simulink model "blance_robot"  (R2024a)
settings: Solver=ode15s  StartTime=0.0  StopTime=15  FixedStep=0.0025  RelTol=1e-3
values from neighbouring files (symbols this model uses):
  K_cons = [-4.92635870386 -6.18040077772 -1.81074270733 -1.19207999822 -32.1009473092 -3.5760389828 4.18688097447 0.16514939939 0.944125254207 0.571537384386 -4.92635870394 -6.18040077751 ... (240 elements, 40x6)]    [K_cons.mat]    (also in k_calc.m = zeros(40,6))
  X = [x1, x2, x1sq, x2sq, x1x2]    [k_calc.m]
undefined symbols (not defined in the file or in its folder): Y, Z
libraries: sm_lib x148, nesl_utility x26, slpidlib x3
(part 1 of 4)
settings Model: Creator=zhuho  LastModifiedBy=zhuho

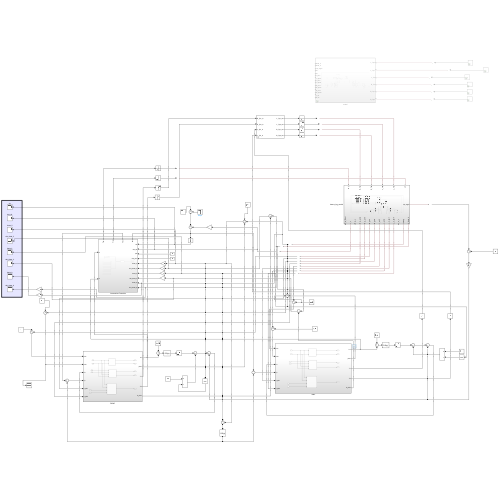
[thumbnail: Simulink's stored preview of the top-level diagram]
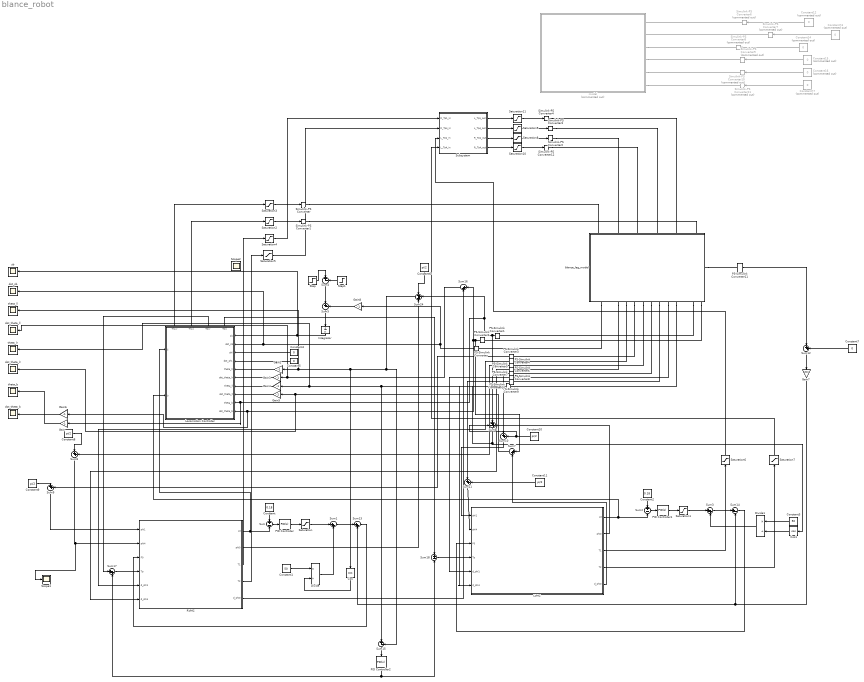
== system blance_robot ==
  Constant : Constant  Value=0.18
  Constant1 : Constant  Value=50
  Constant{6,8..11} (5 alike) : Constant  Value=pi/2
  Constant{12..17} (6 alike) : Constant  Commented=on  Value=0
  Constant2 : Constant  Value=0.18
  Constant3 : Constant  Value=50
  Constant4 : Constant  Value=0
  Constant5 : Constant  Value=0
  Constant7 : Constant  Value=0
  Cos : Trigonometry  Operator=cos
  Cos1 : Trigonometry  Operator=cos
  Divide : Product  Inputs=*/
  Divide1 : Product  Inputs=*/
  Gain{,2..6,8} (7 alike) : Gain  Gain=-1
  Gain7 : Gain  Gain=1500
  Integrator : Integrator
  LVMC : Subsystem
  Locomotion Controller : Subsystem
      settings: PortSchema="{\"entries\":[{\"content\":{\"sides\":[{\"content\":{\"connectorIds\":[\"In1\",\"In2\"]},\"type\":\"ConnectorPlacement.EquallySpacedRectSide\",\"uuid\":\"9f335f1a-920c-489c-ab23-b2605db4f7eb\"},{\"content\":{\"connectorIds\":[\"In3\",\"In4\",\"In5\",\"In6\",\"In7\",\"In8\",\"In9\",\"In10\",\"In11\",\"In12\"],\"side\":\"RIGHT\"},\"type\":\"ConnectorPlacement.EquallySpacedRectSide\",\"uuid\":\"244eb674-a427-495d-a4b5-69ad08e1900d\"},{\"content\":{\"connectorIds\":[\"Out1\",\"Out2\",\"Out3\",\"Out4\"],\"side\":\"TOP\"},\"type\":\"ConnectorPlacement.EquallySpacedRectSide\",\"uuid\":\"a2322f66-0ec6-4fc3-82d4-b6858da1a4af\"}]},\"type\":\"ConnectorPlacement.EquallySpacedConnector\",\"uuid\":\"7ddcb355-7f50-43e9-8496-f4eccb1abc77\"}],\"packageUris\":[\"http://schema.mathworks.com/mf0/Connector/R2020b\"],\"version\":\"1.0\"}"
  PID Controller : slpidlib/PID Controller  Controller=PID  Form=Parallel  TimeDomain=Continuous-time  UseExternalTs=off  SampleTime=-1  IntegratorMethod=Forward Euler  FilterMethod=Forward Euler  ControllerParametersSource=internal  P=500  I=0  UseKiTs=off  D=200  UseExternalDerivativeSource=off  N=100  UseFilter=on  TunerSelectOption=Transfer Function Based (PID Tuner App)  InitialConditionSource=internal  InitialConditionForIntegrator=0  InitialConditionForFilter=0  DifferentiatorICPrevScaledInput=0  ExternalReset=none  TrackingMode=off  Kt=1  LimitOutput=off  SatLimitsSource=internal  UpperSaturationLimit=inf  LowerSaturationLimit=-inf  LinearizeAsGain=on  AntiWindupMode=none  Kb=1  LimitIntegrator=off  UpperIntegratorSaturationLimit=inf  LowerIntegratorSaturationLimit=-inf  POutMin=[]  POutMax=[]  IOutMin=[]  IOutMax=[]  DOutMin=[]  DOutMax=[]  NOutMin=[]  NOutMax=[]  SumOutMin=[]  SumOutMax=[]  SaturationOutMin=[]  SaturationOutMax=[]  PParamMin=[]  PParamMax=[]  IParamMin=[]  IParamMax=[]  DParamMin=[]  DParamMax=[]  NParamMin=[]  NParamMax=[]  KbParamMin=[]  KbParamMax=[]  KtParamMin=[]  KtParamMax=[]  KbOutMin=[]  KbOutMax=[]  KtOutMin=[]  KtOutMax=[]  IntegratorOutMin=[]  IntegratorOutMax=[]  FilterOutMin=[]  FilterOutMax=[]  SumI1OutMin=[]  SumI1OutMax=[]  SumI2OutMin=[]  SumI2OutMax=[]  SumI3OutMin=[]  SumI3OutMax=[]  SumI4OutMin=[]  SumI4OutMax=[]  SumDOutMin=[]  SumDOutMax=[]  DifferentiatorOutMin=[]  DifferentiatorOutMax=[]  FilterDiffOutCoefMin=[]  FilterDiffOutCoefMax=[]  ReciprocalOutMin=[]  ReciprocalOutMax=[]  SumDenOutMin=[]  SumDenOutMax=[]  SumNumOutMin=[]  SumNumOutMax=[]  DivideOutMin=[]  DivideOutMax=[]  UdiffTsProdOutMin=[]  UdiffTsProdOutMax=[]  NTsProdOutMin=[]  NTsProdOutMax=[]  UintegralTsProdOutMin=[]  UintegralTsProdOutMax=[]  UngainTsProdOutMin=[]  UngainTsProdOutMax=[]  ClampingZeroOutDataTypeStr=Inherit: Inherit via back propagation  ClampingZeroOutMin=[]  ClampingZeroOutMax=[]  FilterDenConstantOutDataTypeStr=Inherit: Inherit via back propagation  FilterDenConstantOutMin=[]  FilterDenConstantOutMax=[]  PCopyOutDataTypeStr=Inherit: Inherit via back propagation  PCopyOutMin=[]  PCopyOutMax=[]  NCopyOutDataTypeStr=Inherit: Inherit via back propagation  NCopyOutMin=[]  NCopyOutMax=[]  IntegratorContinuousStateAttributes=''  IntegratorStateMustResolveToSignalObject=off  IntegratorRTWStateStorageClass=Auto  FilterContinuousStateAttributes=''  FilterStateMustResolveToSignalObject=off  FilterRTWStateStorageClass=Auto  ParallelPVariant=InternalParameters  IdealPVariant=Disabled  IVariant=InternalParameters  DVariant=InternalParameters  IntegratorVariant=Continuous  SatVariant=Disabled  AWVariant=Passthrough  PCopyVariant=Disabled  TRVariant=Disabled  FdbkBlocksVariant=Forward  IdealPFdbkVariant=Disabled  SatFdbkVariant=Disabled  DerivativeFilterVariant=ContFilter  NVariant=InternalParameters  NCopyVariant=Disabled  FilterICVariant=InternalICsFilter  IntegratorICVariant=InternalICs  ExternalResetVariant=Disabled  TRSumVariant=Passthrough  SumFdbkVariant=Disabled  SumVariant=Sum_PID  TsampFilterVariant=InternalTs  TsampNgainVariant=Passthrough  TsampIntegralVariant=Disabled_SignalSpec  ExternalSaturationOutDataTypeStr=Inherit: Same as second input  DerivativeSourceVariant=ErrorSignal
  PID Controller1 : slpidlib/PID Controller  Controller=PID  Form=Parallel  TimeDomain=Continuous-time  UseExternalTs=off  SampleTime=-1  IntegratorMethod=Forward Euler  FilterMethod=Forward Euler  ControllerParametersSource=internal  P=500  I=0  UseKiTs=off  D=200  UseExternalDerivativeSource=off  N=100  UseFilter=on  TunerSelectOption=Transfer Function Based (PID Tuner App)  InitialConditionSource=internal  InitialConditionForIntegrator=0  InitialConditionForFilter=0  DifferentiatorICPrevScaledInput=0  ExternalReset=none  TrackingMode=off  Kt=1  LimitOutput=off  SatLimitsSource=internal  UpperSaturationLimit=inf  LowerSaturationLimit=-inf  LinearizeAsGain=on  AntiWindupMode=none  Kb=1  LimitIntegrator=off  UpperIntegratorSaturationLimit=inf  LowerIntegratorSaturationLimit=-inf  POutMin=[]  POutMax=[]  IOutMin=[]  IOutMax=[]  DOutMin=[]  DOutMax=[]  NOutMin=[]  NOutMax=[]  SumOutMin=[]  SumOutMax=[]  SaturationOutMin=[]  SaturationOutMax=[]  PParamMin=[]  PParamMax=[]  IParamMin=[]  IParamMax=[]  DParamMin=[]  DParamMax=[]  NParamMin=[]  NParamMax=[]  KbParamMin=[]  KbParamMax=[]  KtParamMin=[]  KtParamMax=[]  KbOutMin=[]  KbOutMax=[]  KtOutMin=[]  KtOutMax=[]  IntegratorOutMin=[]  IntegratorOutMax=[]  FilterOutMin=[]  FilterOutMax=[]  SumI1OutMin=[]  SumI1OutMax=[]  SumI2OutMin=[]  SumI2OutMax=[]  SumI3OutMin=[]  SumI3OutMax=[]  SumI4OutMin=[]  SumI4OutMax=[]  SumDOutMin=[]  SumDOutMax=[]  DifferentiatorOutMin=[]  DifferentiatorOutMax=[]  FilterDiffOutCoefMin=[]  FilterDiffOutCoefMax=[]  ReciprocalOutMin=[]  ReciprocalOutMax=[]  SumDenOutMin=[]  SumDenOutMax=[]  SumNumOutMin=[]  SumNumOutMax=[]  DivideOutMin=[]  DivideOutMax=[]  UdiffTsProdOutMin=[]  UdiffTsProdOutMax=[]  NTsProdOutMin=[]  NTsProdOutMax=[]  UintegralTsProdOutMin=[]  UintegralTsProdOutMax=[]  UngainTsProdOutMin=[]  UngainTsProdOutMax=[]  ClampingZeroOutDataTypeStr=Inherit: Inherit via back propagation  ClampingZeroOutMin=[]  ClampingZeroOutMax=[]  FilterDenConstantOutDataTypeStr=Inherit: Inherit via back propagation  FilterDenConstantOutMin=[]  FilterDenConstantOutMax=[]  PCopyOutDataTypeStr=Inherit: Inherit via back propagation  PCopyOutMin=[]  PCopyOutMax=[]  NCopyOutDataTypeStr=Inherit: Inherit via back propagation  NCopyOutMin=[]  NCopyOutMax=[]  IntegratorContinuousStateAttributes=''  IntegratorStateMustResolveToSignalObject=off  IntegratorRTWStateStorageClass=Auto  FilterContinuousStateAttributes=''  FilterStateMustResolveToSignalObject=off  FilterRTWStateStorageClass=Auto  ParallelPVariant=InternalParameters  IdealPVariant=Disabled  IVariant=InternalParameters  DVariant=InternalParameters  IntegratorVariant=Continuous  SatVariant=Disabled  AWVariant=Passthrough  PCopyVariant=Disabled  TRVariant=Disabled  FdbkBlocksVariant=Forward  IdealPFdbkVariant=Disabled  SatFdbkVariant=Disabled  DerivativeFilterVariant=ContFilter  NVariant=InternalParameters  NCopyVariant=Disabled  FilterICVariant=InternalICsFilter  IntegratorICVariant=InternalICs  ExternalResetVariant=Disabled  TRSumVariant=Passthrough  SumFdbkVariant=Disabled  SumVariant=Sum_PID  TsampFilterVariant=InternalTs  TsampNgainVariant=Passthrough  TsampIntegralVariant=Disabled_SignalSpec  ExternalSaturationOutDataTypeStr=Inherit: Same as second input  DerivativeSourceVariant=ErrorSignal
  PID Controller2 : slpidlib/PID Controller  Controller=PID  Form=Parallel  TimeDomain=Continuous-time  UseExternalTs=off  SampleTime=-1  IntegratorMethod=Forward Euler  FilterMethod=Forward Euler  ControllerParametersSource=internal  P=300  I=0  UseKiTs=off  D=100  UseExternalDerivativeSource=off  N=100  UseFilter=on  TunerSelectOption=Transfer Function Based (PID Tuner App)  InitialConditionSource=internal  InitialConditionForIntegrator=0  InitialConditionForFilter=0  DifferentiatorICPrevScaledInput=0  ExternalReset=none  TrackingMode=off  Kt=1  LimitOutput=off  SatLimitsSource=internal  UpperSaturationLimit=inf  LowerSaturationLimit=-inf  LinearizeAsGain=on  AntiWindupMode=none  Kb=1  LimitIntegrator=off  UpperIntegratorSaturationLimit=inf  LowerIntegratorSaturationLimit=-inf  POutMin=[]  POutMax=[]  IOutMin=[]  IOutMax=[]  DOutMin=[]  DOutMax=[]  NOutMin=[]  NOutMax=[]  SumOutMin=[]  SumOutMax=[]  SaturationOutMin=[]  SaturationOutMax=[]  PParamMin=[]  PParamMax=[]  IParamMin=[]  IParamMax=[]  DParamMin=[]  DParamMax=[]  NParamMin=[]  NParamMax=[]  KbParamMin=[]  KbParamMax=[]  KtParamMin=[]  KtParamMax=[]  KbOutMin=[]  KbOutMax=[]  KtOutMin=[]  KtOutMax=[]  IntegratorOutMin=[]  IntegratorOutMax=[]  FilterOutMin=[]  FilterOutMax=[]  SumI1OutMin=[]  SumI1OutMax=[]  SumI2OutMin=[]  SumI2OutMax=[]  SumI3OutMin=[]  SumI3OutMax=[]  SumI4OutMin=[]  SumI4OutMax=[]  SumDOutMin=[]  SumDOutMax=[]  DifferentiatorOutMin=[]  DifferentiatorOutMax=[]  FilterDiffOutCoefMin=[]  FilterDiffOutCoefMax=[]  ReciprocalOutMin=[]  ReciprocalOutMax=[]  SumDenOutMin=[]  SumDenOutMax=[]  SumNumOutMin=[]  SumNumOutMax=[]  DivideOutMin=[]  DivideOutMax=[]  UdiffTsProdOutMin=[]  UdiffTsProdOutMax=[]  NTsProdOutMin=[]  NTsProdOutMax=[]  UintegralTsProdOutMin=[]  UintegralTsProdOutMax=[]  UngainTsProdOutMin=[]  UngainTsProdOutMax=[]  ClampingZeroOutDataTypeStr=Inherit: Inherit via back propagation  ClampingZeroOutMin=[]  ClampingZeroOutMax=[]  FilterDenConstantOutDataTypeStr=Inherit: Inherit via back propagation  FilterDenConstantOutMin=[]  FilterDenConstantOutMax=[]  PCopyOutDataTypeStr=Inherit: Inherit via back propagation  PCopyOutMin=[]  PCopyOutMax=[]  NCopyOutDataTypeStr=Inherit: Inherit via back propagation  NCopyOutMin=[]  NCopyOutMax=[]  IntegratorContinuousStateAttributes=''  IntegratorStateMustResolveToSignalObject=off  IntegratorRTWStateStorageClass=Auto  FilterContinuousStateAttributes=''  FilterStateMustResolveToSignalObject=off  FilterRTWStateStorageClass=Auto  ParallelPVariant=InternalParameters  IdealPVariant=Disabled  IVariant=InternalParameters  DVariant=InternalParameters  IntegratorVariant=Continuous  SatVariant=Disabled  AWVariant=Passthrough  PCopyVariant=Disabled  TRVariant=Disabled  FdbkBlocksVariant=Forward  IdealPFdbkVariant=Disabled  SatFdbkVariant=Disabled  DerivativeFilterVariant=ContFilter  NVariant=InternalParameters  NCopyVariant=Disabled  FilterICVariant=InternalICsFilter  IntegratorICVariant=InternalICs  ExternalResetVariant=Disabled  TRSumVariant=Passthrough  SumFdbkVariant=Disabled  SumVariant=Sum_PID  TsampFilterVariant=InternalTs  TsampNgainVariant=Passthrough  TsampIntegralVariant=Disabled_SignalSpec  ExternalSaturationOutDataTypeStr=Inherit: Same as second input  DerivativeSourceVariant=ErrorSignal
  PS-Simulink Converter{,1..11} (12 alike) : nesl_utility/PS-Simulink Converter  PhysicalDomain=network_engine_domain  SubClassName=ps_output  LeftPortType=input  RightPortType=output  PseudoPeriodic=off  Frequencies=[]  VectorFormat=inherit  Unit=inherit  AffineConversion=off
  RVMC : Subsystem
  Saturation : Saturate  UpperLimit=9  LowerLimit=-9
  Saturation1 : Saturate  UpperLimit=9  LowerLimit=-9
  Saturation{8..11} (4 alike) : Saturate  UpperLimit=100  LowerLimit=-100
  Saturation{2..7} (6 alike) : Saturate  UpperLimit=10  LowerLimit=-10
  Scope1 : Scope
  Simulink-PS Converter{,1..4,12} (6 alike) : nesl_utility/Simulink-PS Converter  PhysicalDomain=network_engine_domain  SubClassName=ps_input  LeftPortType=input  RightPortType=output  PseudoPeriodic=off  Frequencies=[]  NoiseDistribution=none  NoiseParameters=[]  Unit=1  AffineConversion=off  FilteringAndDerivatives=provide  SimscapeFilterOrder=1  InputFilterTimeConstant=0.001  UdotUserProvided=0
  Simulink-PS Converter{6..11} (6 alike) : nesl_utility/Simulink-PS Converter  Commented=on  PhysicalDomain=network_engine_domain  SubClassName=ps_input  LeftPortType=input  RightPortType=output  PseudoPeriodic=off  Frequencies=[]  NoiseDistribution=none  NoiseParameters=[]  Unit=1  AffineConversion=off  FilteringAndDerivatives=provide  SimscapeFilterOrder=1  InputFilterTimeConstant=0.001  UdotUserProvided=0
  Step : Step  Time=0.8  After=-2.5  SampleTime=0
  Step1 : Step  Time=5  After=-2.5  SampleTime=0
  Subsystem : Subsystem  mask{Jump_time=4.3, Jump_torque=10}
      mask DialogControl ParameterGroupVar Prompt: 参数
  Sum : Sum  Inputs=+|-
  Sum{1,3,7..13,16..17} (11 alike) : Sum  Inputs=|++
  Sum{4..5,14..15} (4 alike) : Sum  Inputs=|+-
  Sum18 : Sum  Inputs=+|-
  Sum2 : Sum  Inputs=+|-
  Sum24 : Sum  Inputs=-++
  Sum6 : Sum  Inputs=-++
  blance_leg_model : Subsystem
      settings: PortSchema="{\"entries\":[{\"content\":{\"sides\":[{\"content\":{\"connectorIds\":[\"LConn1\",\"LConn2\",\"LConn3\",\"LConn4\",\"LConn5\",\"LConn6\"]},\"type\":\"ConnectorPlacement.EquallySpacedRectSide\",\"uuid\":\"ed635f35-0836-4900-93e3-56fc3520c8de\"},{\"content\":{\"connectorIds\":[\"RConn1\",\"RConn2\",\"RConn3\",\"RConn4\",\"RConn5\",\"RConn6\",\"RConn7\",\"RConn8\",\"RConn9\",\"RConn10\",\"RConn11\",\"RConn12\",\"RConn13\",\"RConn14\"],\"side\":\"RIGHT\"},\"type\":\"ConnectorPlacement.EquallySpacedRectSide\",\"uuid\":\"bb235ec0-defd-4ad9-96f6-8533dab3fbd9\"},{\"content\":{\"connectorIds\":[],\"side\":\"TOP\"},\"type\":\"ConnectorPlacement.EquallySpacedRectSide\",\"uuid\":\"d719db37-8b3a-4344-b330-944fde418334\"},{\"content\":{\"connectorIds\":[\"RConn15\"],\"side\":\"BOTTOM\"},\"type\":\"ConnectorPlacement.EquallySpacedRectSide\",\"uuid\":\"20f9270b-6ab1-4e89-bf00-e838d12c3c13\"}]},\"type\":\"ConnectorPlacement.EquallySpacedConnector\",\"uuid\":\"a2f25b71-0047-4a2d-a238-dad76f034ab1\"}],\"packageUris\":[\"http://schema.mathworks.com/mf0/Connector/R2020b\"],\"version\":\"1.0\"}"
  dot_sb : Scope
  dot_theta_b : Scope
  dot_theta_ll : Scope
  dot_theta_lr : Scope
  model : Subsystem  Commented=on
  sb : Scope
  theta_b : Scope
  theta_ll : Scope
  theta_lr : Scope
  Scope2 : Scope
  wires:
  Constant/1 -> Sum/1
  Sum/1 -> PID Controller/1
  PID Controller/1 -> Saturation/1
  Saturation/1 -> Sum1/1
  Constant2/1 -> Sum2/1
  Sum2/1 -> PID Controller1/1
  PID Controller1/1 -> Saturation1/1
  Saturation1/1 -> Sum3/1
  RVMC/1(L0) -> Locomotion Controller/1(ll), Sum/2
  LVMC/1(L0) -> Locomotion Controller/2(lr), Sum2/2
  Locomotion Controller/1(Tlw,r) -> Saturation3/1
  Locomotion Controller/2(Tlw,l) -> Saturation2/1
  Saturation2/1 -> Simulink-PS Converter1/1
  Saturation3/1 -> Simulink-PS Converter/1
  Step/1 -> Sum4/1
  Step1/1 -> Sum4/2
  Sum4/1 -> Sum5/1
  Sum5/1 -> Integrator/1
  PS-Simulink Converter/1 -> Gain8/1, dot_sb/1, Locomotion Controller/4(dot_sb)
  Constant4/1 -> Locomotion Controller/5(phi)
  Constant5/1 -> Locomotion Controller/6(dot_phi.)
  Constant6/1 -> Sum24/1
  RVMC/2(phi0) -> Sum24/3
  Sum24/1 -> Sum15/2, theta_ll/1, Gain2/1, Cos/1
  RVMC/5(d_phi0) -> Sum16/2
  Sum16/1 -> dot_theta_ll/1, Gain3/1
  Constant10/1 -> Sum6/1, Sum10/2
  LVMC/2(phi0) -> Sum6/3
  LVMC/5(d_phi0) -> Sum7/2
  Sum6/1 -> Cos1/1, theta_lr/1, Gain4/1, Sum15/1
  Sum7/1 -> dot_theta_lr/1, Gain5/1
  PS-Simulink Converter5/1 -> Sum8/2
  Constant8/1 -> Sum8/1
  Sum8/1 -> Scope1/1, RVMC/2(phi4)
  PS-Simulink Converter6/1 -> RVMC/6(d_phi4)
  Constant9/1 -> Sum9/1
  PS-Simulink Converter4/1 -> RVMC/5(d_phi1)
  PS-Simulink Converter7/1 -> Sum10/1
  Sum10/1 -> LVMC/1(phi1)
  PS-Simulink Converter8/1 -> LVMC/5(d_phi1)
  PS-Simulink Converter9/1 -> Sum11/1
  Constant11/1 -> Sum11/2
  Sum11/1 -> LVMC/2(phi4)
  PS-Simulink Converter10/1 -> LVMC/6(d_phi4)
  RVMC/4(T2) -> Saturation5/1
  RVMC/3(T1) -> Saturation4/1
  LVMC/3(T1) -> Saturation6/1
  LVMC/4(T2) -> Saturation7/1
  PS-Simulink Converter3/1 -> Sum9/2
  Sum9/1 -> RVMC/1(phi1)
  Constant12/1 -> Simulink-PS Converter6/1
  Constant13/1 -> Simulink-PS Converter7/1
  Constant14/1 -> Simulink-PS Converter8/1
  Constant15/1 -> Simulink-PS Converter9/1
  Constant16/1 -> Simulink-PS Converter10/1
  Constant17/1 -> Simulink-PS Converter11/1
  Integrator/1 -> Locomotion Controller/3(sb), sb/1
  Gain2/1 -> Locomotion Controller/7(theta_lr)
  Gain3/1 -> Locomotion Controller/8(dot_theta_lr)
  Gain4/1 -> Locomotion Controller/9(theta_ll)
  Gain5/1 -> Locomotion Controller/10(dot_theta_ll)
  PS-Simulink Converter1/1 -> Gain/1, Locomotion Controller/11(theta_b), Sum24/2, Sum6/2
  PS-Simulink Converter2/1 -> Sum7/1, Gain6/1, Locomotion Controller/12(dot_theta_b), Sum16/1
  Gain/1 -> theta_b/1
  Gain6/1 -> dot_theta_b/1
  Constant1/1 -> Divide/1
  Cos/1 -> Divide/2
  Divide/1 -> Sum1/2
  Constant3/1 -> Divide1/1
  Cos1/1 -> Divide1/2
  Divide1/1 -> Sum3/2
  PS-Simulink Converter11/1 -> Sum12/1
  Constant7/1 -> Sum12/2
  Sum12/1 -> Gain7/1
  Sum1/1 -> Sum13/1
  Gain7/1 -> Sum14/2, Sum13/2
  Sum13/1 -> RVMC/3(F0)
  Sum3/1 -> Sum14/1
  Sum14/1 -> LVMC/3(F0)
  Gain8/1 -> Sum5/2
  Sum15/1 -> PID Controller2/1
  PID Controller2/1 -> Sum17/2, Sum18/2
  Locomotion Controller/3(Tbl,r) -> Sum17/1
  Sum17/1 -> RVMC/4(Tp)
  Sum18/1 -> LVMC/4(Tp)
  Locomotion Controller/4(Tbl,l) -> Sum18/1
  Saturation4/1 -> Subsystem/1(R_Tp1_in)
  Subsystem/3(R_Tp1_out) -> Saturation8/1
  Saturation8/1 -> Simulink-PS Converter2/1
  Saturation5/1 -> Subsystem/2(R_Tp4_in)
  Subsystem/2(L_Tp4_out) -> Saturation9/1
  Saturation9/1 -> Simulink-PS Converter3/1
  Subsystem/4(R_Tp4_out) -> Saturation10/1
  Saturation10/1 -> Simulink-PS Converter12/1
  Saturation6/1 -> Subsystem/3(L_Tp1_in)
  Subsystem/1(L_Tp1_out) -> Saturation11/1
  Saturation11/1 -> Simulink-PS Converter4/1
  Saturation7/1 -> Subsystem/4(L_Tp4_in)
  connections:
  Simulink-PS Converter6/RConn1 -- model/LConn1
  Simulink-PS Converter7/RConn1 -- model/LConn2
  model/LConn3 -- Simulink-PS Converter8/RConn1
  model/LConn4 -- Simulink-PS Converter9/RConn1
  model/LConn5 -- Simulink-PS Converter10/RConn1
  model/LConn6 -- Simulink-PS Converter11/RConn1
  blance_leg_model/RConn13 -- PS-Simulink Converter1/LConn1
  blance_leg_model/RConn14 -- PS-Simulink Converter2/LConn1
  blance_leg_model/RConn2 -- PS-Simulink Converter/LConn1
  blance_leg_model/RConn6 -- PS-Simulink Converter3/LConn1
  blance_leg_model/RConn5 -- PS-Simulink Converter4/LConn1
  blance_leg_model/RConn7 -- PS-Simulink Converter5/LConn1
  blance_leg_model/RConn4 -- PS-Simulink Converter6/LConn1
  blance_leg_model/RConn8 -- PS-Simulink Converter7/LConn1
  blance_leg_model/RConn10 -- PS-Simulink Converter8/LConn1
  blance_leg_model/RConn9 -- PS-Simulink Converter9/LConn1
  blance_leg_model/RConn11 -- PS-Simulink Converter10/LConn1
  blance_leg_model/RConn15 -- PS-Simulink Converter11/LConn1
  Simulink-PS Converter/RConn1 -- blance_leg_model/LConn1
  Simulink-PS Converter1/RConn1 -- blance_leg_model/LConn6
  Simulink-PS Converter2/RConn1 -- blance_leg_model/LConn2
  Simulink-PS Converter12/RConn1 -- blance_leg_model/LConn3
  Simulink-PS Converter4/RConn1 -- blance_leg_model/LConn5
  Simulink-PS Converter3/RConn1 -- blance_leg_model/LConn4

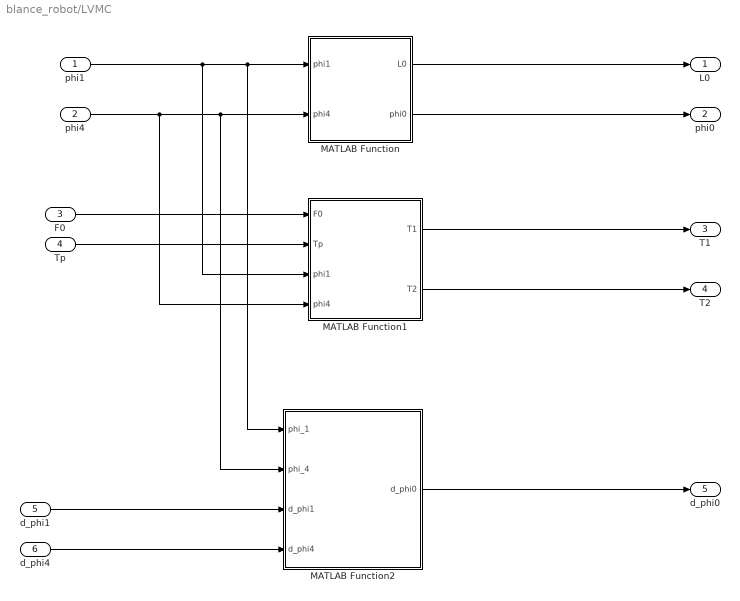
== system blance_robot/LVMC ==
  phi1 : Inport
  phi4 : Inport  Port=2
  F0 : Inport  Port=3
  Tp : Inport  Port=4
  d_phi1 : Inport  Port=5
  d_phi4 : Inport  Port=6
  MATLAB Function : MATLAB Function  TreatAsAtomicUnit=on
  MATLAB Function1 : MATLAB Function  TreatAsAtomicUnit=on
  MATLAB Function2 : MATLAB Function  TreatAsAtomicUnit=on
  L0 : Outport
  phi0 : Outport  Port=2
  T1 : Outport  Port=3
  T2 : Outport  Port=4
  d_phi0 : Outport  Port=5
  wires:
  phi1/1 -> MATLAB Function1/3(phi1), MATLAB Function2/1(phi_1), MATLAB Function/1(phi1)
  phi4/1 -> MATLAB Function1/4(phi4), MATLAB Function2/2(phi_4), MATLAB Function/2(phi4)
  F0/1 -> MATLAB Function1/1(F0)
  Tp/1 -> MATLAB Function1/2(Tp)
  d_phi1/1 -> MATLAB Function2/3(d_phi1)
  d_phi4/1 -> MATLAB Function2/4(d_phi4)
  MATLAB Function/1(L0) -> L0/1
  MATLAB Function/2(phi0) -> phi0/1
  MATLAB Function1/1(T1) -> T1/1
  MATLAB Function1/2(T2) -> T2/1
  MATLAB Function2/1(d_phi0) -> d_phi0/1

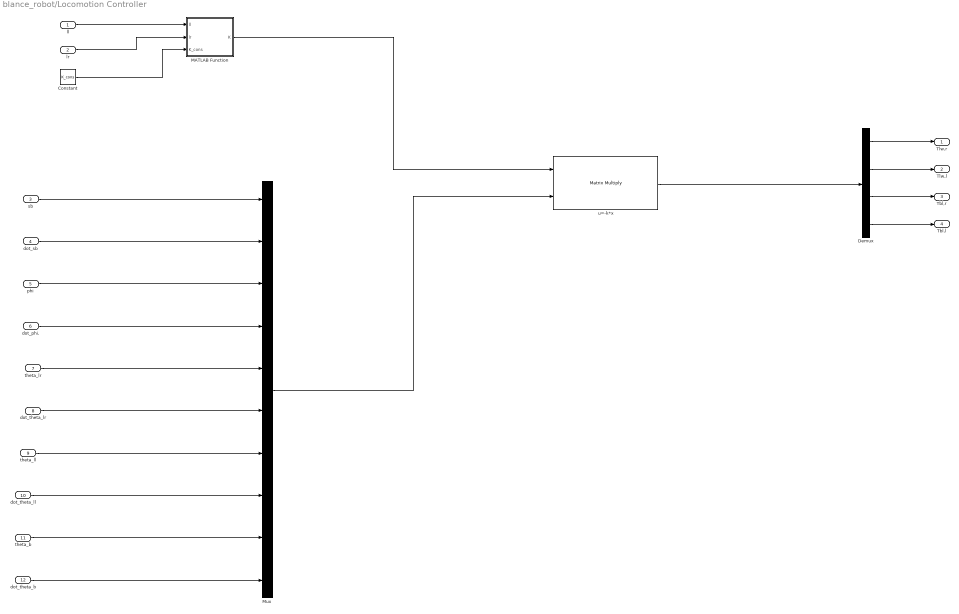
== system blance_robot/Locomotion Controller ==
  ll : Inport
  lr : Inport  Port=2
  sb : Inport  Port=3
  dot_sb : Inport  Port=4
  phi : Inport  Port=5
  dot_phi. : Inport  Port=6
  theta_lr : Inport  Port=7
  dot_theta_lr : Inport  Port=8
  theta_ll : Inport  Port=9
  dot_theta_ll : Inport  Port=10
  theta_b : Inport  Port=11
  dot_theta_b : Inport  Port=12
  Constant : Constant  Value=K_cons
  Demux : Demux
  MATLAB Function : MATLAB Function  TreatAsAtomicUnit=on
  Mux : Mux  Inputs=10
  u=-k*x : Product  Multiplication=Matrix(*)
  Tlw,r : Outport
  Tlw,l : Outport  Port=2
  Tbl,r : Outport  Port=3
  Tbl,l : Outport  Port=4
  wires:
  ll/1 -> MATLAB Function/1(ll)
  lr/1 -> MATLAB Function/2(lr)
  Constant/1 -> MATLAB Function/3(K_cons)
  sb/1 -> Mux/1
  dot_sb/1 -> Mux/2
  phi/1 -> Mux/3
  dot_phi./1 -> Mux/4
  theta_lr/1 -> Mux/5
  dot_theta_lr/1 -> Mux/6
  theta_ll/1 -> Mux/7
  dot_theta_ll/1 -> Mux/8
  theta_b/1 -> Mux/9
  dot_theta_b/1 -> Mux/10
  MATLAB Function/1(K) -> u=-k*x/1
  Mux/1 -> u=-k*x/2
  u=-k*x/1 -> Demux/1
  Demux/1 -> Tlw,r/1
  Demux/2 -> Tlw,l/1
  Demux/3 -> Tbl,r/1
  Demux/4 -> Tbl,l/1

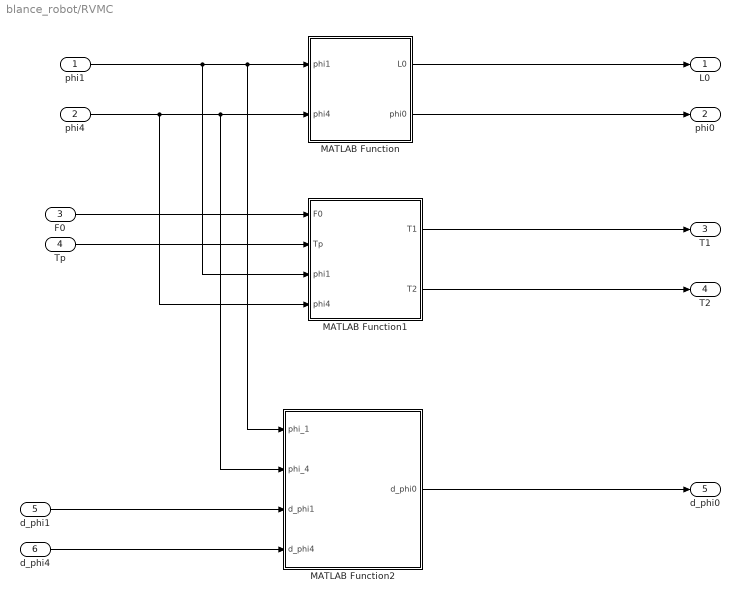
== system blance_robot/RVMC ==
  phi1 : Inport
  phi4 : Inport  Port=2
  F0 : Inport  Port=3
  Tp : Inport  Port=4
  d_phi1 : Inport  Port=5
  d_phi4 : Inport  Port=6
  MATLAB Function : MATLAB Function  TreatAsAtomicUnit=on
  MATLAB Function1 : MATLAB Function  TreatAsAtomicUnit=on
  MATLAB Function2 : MATLAB Function  TreatAsAtomicUnit=on
  L0 : Outport
  phi0 : Outport  Port=2
  T1 : Outport  Port=3
  T2 : Outport  Port=4
  d_phi0 : Outport  Port=5
  wires:
  phi1/1 -> MATLAB Function1/3(phi1), MATLAB Function2/1(phi_1), MATLAB Function/1(phi1)
  phi4/1 -> MATLAB Function1/4(phi4), MATLAB Function2/2(phi_4), MATLAB Function/2(phi4)
  F0/1 -> MATLAB Function1/1(F0)
  Tp/1 -> MATLAB Function1/2(Tp)
  d_phi1/1 -> MATLAB Function2/3(d_phi1)
  d_phi4/1 -> MATLAB Function2/4(d_phi4)
  MATLAB Function/1(L0) -> L0/1
  MATLAB Function/2(phi0) -> phi0/1
  MATLAB Function1/1(T1) -> T1/1
  MATLAB Function1/2(T2) -> T2/1
  MATLAB Function2/1(d_phi0) -> d_phi0/1

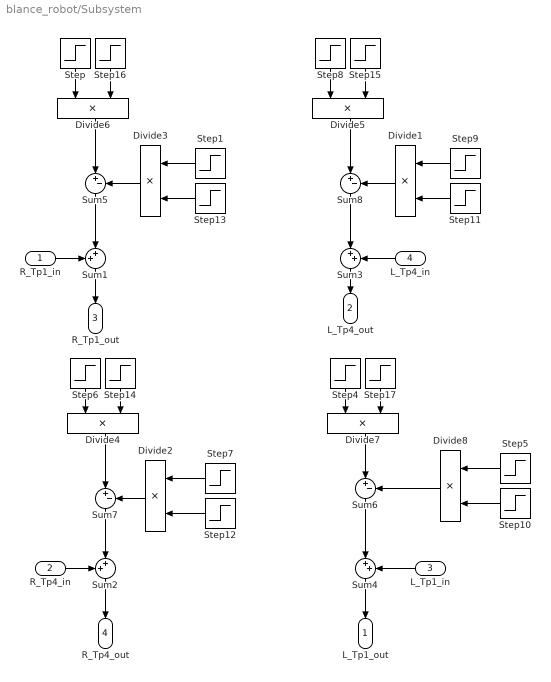
== system blance_robot/Subsystem ==
  R_Tp1_in : Inport
  R_Tp4_in : Inport  Port=2
  L_Tp1_in : Inport  Port=3
  L_Tp4_in : Inport  Port=4
  Divide{1..8} (8 alike) : Product  Inputs=**
  Step : Step  Time=Jump_time  After=-Jump_torque  SampleTime=0
  Step1 : Step  Time=Jump_time+0.15  After=-Jump_torque  SampleTime=0
  Step{10..13} (4 alike) : Step  Time=Jump_time+0.4  Before=1  After=0  SampleTime=0
  Step{14..17} (4 alike) : Step  Time=Jump_time+0.2  Before=1  After=0  SampleTime=0
  Step4 : Step  Time=Jump_time  After=-Jump_torque  SampleTime=0
  Step5 : Step  Time=Jump_time+0.15  After=-Jump_torque  SampleTime=0
  Step6 : Step  Time=Jump_time  After=Jump_torque  SampleTime=0
  Step7 : Step  Time=Jump_time+0.15  After=Jump_torque  SampleTime=0
  Step8 : Step  Time=Jump_time  After=Jump_torque  SampleTime=0
  Step9 : Step  Time=Jump_time+0.15  After=Jump_torque  SampleTime=0
  Sum1 : Sum  Inputs=++|
  Sum2 : Sum  Inputs=++|
  Sum3 : Sum  Inputs=|++
  Sum4 : Sum  Inputs=|++
  Sum{5..8} (4 alike) : Sum  Inputs=|+-
  L_Tp1_out : Outport
  L_Tp4_out : Outport  Port=2
  R_Tp1_out : Outport  Port=3
  R_Tp4_out : Outport  Port=4
  wires:
  Step9/1 -> Divide1/1
  Divide6/1 -> Sum5/1
  Step14/1 -> Divide4/2
  Step5/1 -> Divide8/1
  R_Tp1_in/1 -> Sum1/1
  Sum1/1 -> R_Tp1_out/1
  Step4/1 -> Divide7/1
  Divide1/1 -> Sum8/2
  Divide5/1 -> Sum8/1
  Step/1 -> Divide6/1
  Step17/1 -> Divide7/2
  Step6/1 -> Divide4/1
  Sum3/1 -> L_Tp4_out/1
  Step15/1 -> Divide5/2
  Sum2/1 -> R_Tp4_out/1
  Sum4/1 -> L_Tp1_out/1
  R_Tp4_in/1 -> Sum2/1
  Divide7/1 -> Sum6/1
  Sum5/1 -> Sum1/2
  Step10/1 -> Divide8/2
  L_Tp4_in/1 -> Sum3/2
  Step12/1 -> Divide2/2
  Step13/1 -> Divide3/2
  Divide2/1 -> Sum7/2
  Step11/1 -> Divide1/2
  Sum8/1 -> Sum3/1
  Divide8/1 -> Sum6/2
  Step8/1 -> Divide5/1
  Sum7/1 -> Sum2/2
  Divide4/1 -> Sum7/1
  L_Tp1_in/1 -> Sum4/2
  Step7/1 -> Divide2/1
  Step1/1 -> Divide3/1
  Divide3/1 -> Sum5/2
  Sum6/1 -> Sum4/1
  Step16/1 -> Divide6/2
